simulink library "variableAltitudeBasisParams_cl"  (R2020a)
settings: Solver=VariableStepAuto  StartTime=0.0  StopTime=10.0  RelTol=1e-3
undefined symbols (not defined in the file or in its folder): el, fltCtrl, HILVLCONTROLLER, hiLvlCtrl, initializeBussesFromBlock
settings Model: Creator=mcobb  LastModifiedBy=John Jr
settings DataIOCC: ReturnWorkspaceOutputs=off
settings DebuggingCC: ArithmeticOperatorsInVariantConditions=warning
settings SFSimCC: CustomCodeUndefinedFunction=UseInterfaceOnly

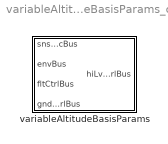
== system variableAltitudeBasisParams_cl ==
  variableAltitudeBasisParams : Subsystem  LoadFcn=initializeBussesFromBlock(gcb)  InitFcn=initializeBussesFromBlock(gcb)  StartFcn=initializeBussesFromBlock(gcb)  VariantControl=strcmpi(HILVLCONTROLLER,'variableAltitudeBasisParams')  mask{basisParams=hiLvlCtrl.basisParams.Value}
      mask prompts: basisParams "Basis Parameters"

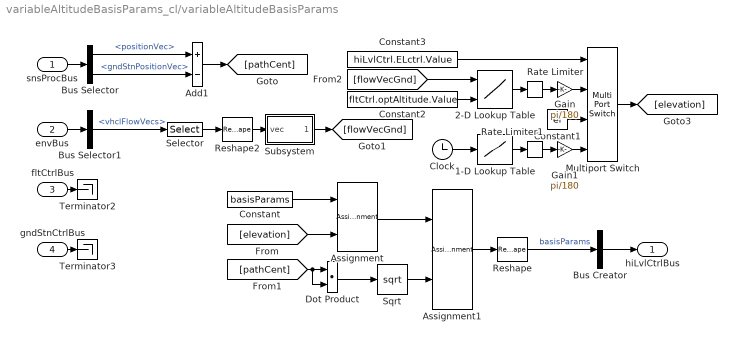
== system variableAltitudeBasisParams_cl/variableAltitudeBasisParams ==
  snsProcBus : Inport  OutDataTypeStr=Bus: sensorsProcessingBus
  envBus : Inport  Port=2  OutDataTypeStr=Bus: envBus
  fltCtrlBus : Inport  Port=3  OutDataTypeStr=Bus: fltCtrlBus
  gndStnCtrlBus : Inport  Port=4  OutDataTypeStr=Bus: gndStnCtrlBus
  1-D Lookup Table : Lookup_n-D  NumberOfTableDimensions=1  BreakpointsForDimension1=[0 500 1500]  Table=[el*180/pi 15 40]  InterpMethod=Flat  InternalRulePriority=Speed  RndMeth=Simplest  InputSameDT=on
  2-D Lookup Table : Lookup_n-D  BreakpointsForDimension1=hiLvlCtrl.velRef.Value  BreakpointsForDimension2=hiLvlCtrl.altRef.Value  Table=hiLvlCtrl.elevationLookup.Value  InternalRulePriority=Speed  RndMeth=Simplest  InputSameDT=on
  Add1 : Sum  Inputs=+-
  Assignment : Assignment  DiagnosticForDimensions=Warning  IndexOptions=Index vector (dialog)  Indices=3  OutputSizes=1
  Assignment1 : Assignment  DiagnosticForDimensions=Warning  IndexOptions=Index vector (dialog)  Indices=5  OutputSizes=1
  Bus Creator : BusCreator  Inputs=1  OutDataTypeStr=Bus: hiLvlCtrlBus
  Bus Selector : BusSelector  OutputSignals=positionVec,gndStnPositionVec
  Bus Selector1 : BusSelector  OutputSignals=vhclFlowVecs
  Clock : Clock
  Constant : Constant  Value=basisParams
  Constant1 : Constant  Value=el
  Constant2 : Constant  Value=fltCtrl.optAltitude.Value
  Constant3 : Constant  Value=hiLvlCtrl.ELctrl.Value
  Dot Product : DotProduct  InputSameDT=on  OutDataTypeStr=Inherit: Inherit via internal rule
  Gain : Gain  Gain=pi/180
  Gain1 : Gain  Gain=pi/180
  Multiport Switch : MultiPortSwitch  DataPortOrder=Specify indices  Inputs=2  DataPortIndices={0,1,2}
  Rate Limiter : RateLimiter  RisingSlewLimit=hiLvlCtrl.ELslew.Value  FallingSlewLimit=-hiLvlCtrl.ELslew.Value  SampleTimeMode=inherited
  Rate Limiter1 : RateLimiter  RisingSlewLimit=hiLvlCtrl.ELslew.Value  FallingSlewLimit=-hiLvlCtrl.ELslew.Value  SampleTimeMode=inherited
  Reshape : Reshape  OutputDimensionality=Column vector (2-D)
  Reshape2 : Reshape  OutputDimensionality=Column vector (2-D)
  Selector : Selector  NumberOfDimensions=2  InputPortWidth=3  IndexOptions=Select all,Index vector (dialog)  Indices=[1 3],5  OutputSizes=1,1
  Sqrt : Sqrt  SaturateOnIntegerOverflow=on
  Subsystem : Subsystem
  Terminator2 : Terminator
  Terminator3 : Terminator
  hiLvlCtrlBus : Outport  OutDataTypeStr=Bus: hiLvlCtrlBus  VectorParamsAs1DForOutWhenUnconnected=off
  wires:
  Assignment1/1 -> Reshape/1
  Assignment/1 -> Assignment1/1
  Sqrt/1 -> Assignment1/2
  Bus Selector/2 -> Add1/2  "<gndStnPositionVec>"
  Bus Selector/1 -> Add1/1  "<positionVec>"
  Dot Product/1 -> Sqrt/1
  envBus/1 -> Bus Selector1/1
  gndStnCtrlBus/1 -> Terminator3/1
  Bus Creator/1 -> hiLvlCtrlBus/1
  Constant/1 -> Assignment/1
  fltCtrlBus/1 -> Terminator2/1
  snsProcBus/1 -> Bus Selector/1
  Reshape/1 -> Bus Creator/1  "basisParams"
  [elevation] -> Assignment/2
  [pathCent] -> Dot Product/2, Dot Product/1
  Add1/1 -> [pathCent]
  Selector/1 -> Reshape2/1
  Bus Selector1/1 -> Selector/1  "<vhclFlowVecs>"
  Constant1/1 -> Multiport Switch/3
  2-D Lookup Table/1 -> Rate Limiter/1
  Multiport Switch/1 -> [elevation]
  Constant3/1 -> Multiport Switch/1
  Gain/1 -> Multiport Switch/2
  Rate Limiter/1 -> Gain/1
  [flowVecGnd] -> 2-D Lookup Table/1
  Constant2/1 -> 2-D Lookup Table/2
  Rate Limiter1/1 -> Gain1/1
  Gain1/1 -> Multiport Switch/4
  Reshape2/1 -> Subsystem/1(vec)
  Subsystem/1(norm) -> [flowVecGnd]
  1-D Lookup Table/1 -> Rate Limiter1/1
  Clock/1 -> 1-D Lookup Table/1

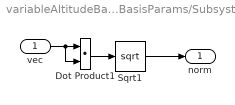
== system variableAltitudeBasisParams_cl/variableAltitudeBasisParams/Subsystem ==
  vec : Inport
  Dot Product1 : DotProduct  InputSameDT=on  OutDataTypeStr=Inherit: Inherit via internal rule
  Sqrt1 : Sqrt  SaturateOnIntegerOverflow=on
  norm : Outport
  wires:
  Dot Product1/1 -> Sqrt1/1
  vec/1 -> Dot Product1/2, Dot Product1/1
  Sqrt1/1 -> norm/1
